simulink model "model_1"  (R2025b)
settings: Solver=VariableStepAuto  StartTime=0.0  StopTime=10.0  RelTol=1e-3
settings Model: Creator=CDA1GA  LastModifiedBy=CDA1GA

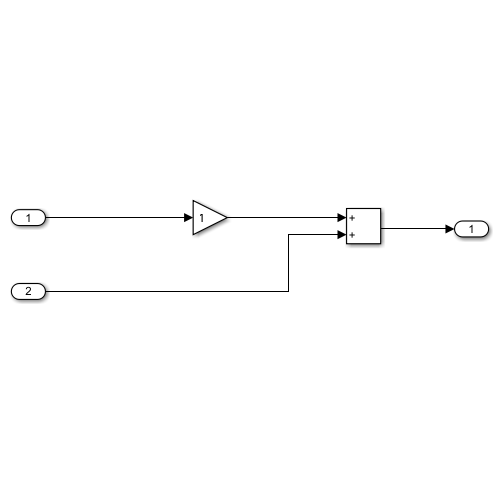
[thumbnail: Simulink's stored preview of the top-level diagram]
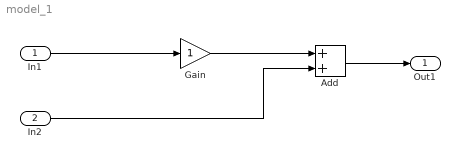
== system model_1 ==
  In1 : Inport
  In2 : Inport  Port=2
  Add : Sum
  Gain : Gain
  Out1 : Outport
  wires:
  Gain/1 -> Add/1
  In1/1 -> Gain/1
  In2/1 -> Add/2
  Add/1 -> Out1/1
